simulink model "centre_out_with_two_joint_arm"  (R2021a)
settings: Solver=VariableStepAuto  StartTime=0.0  StopTime=inf  RelTol=1e-3
libraries: vrlib x1
settings Model: Creator=kbhar  LastModifiedBy=kbhar

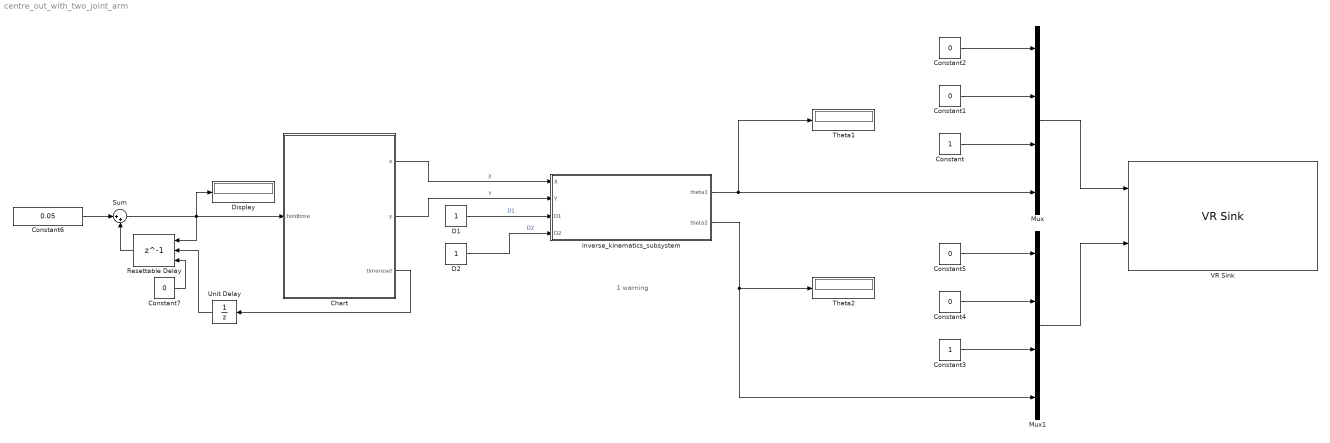
== system centre_out_with_two_joint_arm ==
  note: 1 warning
  Chart : Stateflow chart  TreatAsAtomicUnit=on
  Constant : Constant
  Constant{1..2,4..5,7} (5 alike) : Constant  Value=0
  Constant3 : Constant
  Constant6 : Constant  Value=0.05
  D1 : Constant
  D2 : Constant
  Display : Display
  Mux : Mux
  Mux1 : Mux
  Resettable Delay : Delay  DelayLength=1  InitialConditionSource=Input port  ExternalReset=Rising
      settings: InputPortMap=u0,r5,p4
  Sum : Sum  Inputs=|++
  Theta1 : Display
  Theta2 : Display
  Unit Delay : UnitDelay  SampleTime=-1  HasFrameUpgradeWarning=on
  VR Sink : vrlib/VR Sink  InstantiateOnLoad=on  SampleTime=0.1  ViewEnable=on  RemoteChange=off  RemoteView=off  FieldsWritten=shoulder_joint.rotation.4.1.1.double#elbow_joint.rotation.4.1.1.double  WorldFileName=C:\Bharat\College\Projects\Arm Control\Files\test_two_joint_arm.wrl  AutoView=off  VideoDimensions=[]  AllowVariableSize=off
  inverse_kinematics_subsystem : Subsystem
  wires:
  inverse_kinematics_subsystem/2(theta2) -> Mux1/4, Theta2/1
  inverse_kinematics_subsystem/1(theta1) -> Mux/4, Theta1/1
  Constant2/1 -> Mux/1
  Constant/1 -> Mux/3
  Constant4/1 -> Mux1/2
  Constant3/1 -> Mux1/3
  Constant5/1 -> Mux1/1
  Mux1/1 -> VR Sink/2
  Mux/1 -> VR Sink/1
  Constant1/1 -> Mux/2
  Chart/3(timereset) -> Unit Delay/1
  Constant6/1 -> Sum/1
  Resettable Delay/1 -> Sum/2
  Sum/1 -> Resettable Delay/1, Chart/1(holdtime), Display/1
  Unit Delay/1 -> Resettable Delay/2
  Chart/1(x) -> inverse_kinematics_subsystem/1(X)  "X"
  Chart/2(y) -> inverse_kinematics_subsystem/2(Y)  "Y"
  D1/1 -> inverse_kinematics_subsystem/3(D1)  "D1"
  D2/1 -> inverse_kinematics_subsystem/4(D2)  "D2"
  Constant7/1 -> Resettable Delay/3

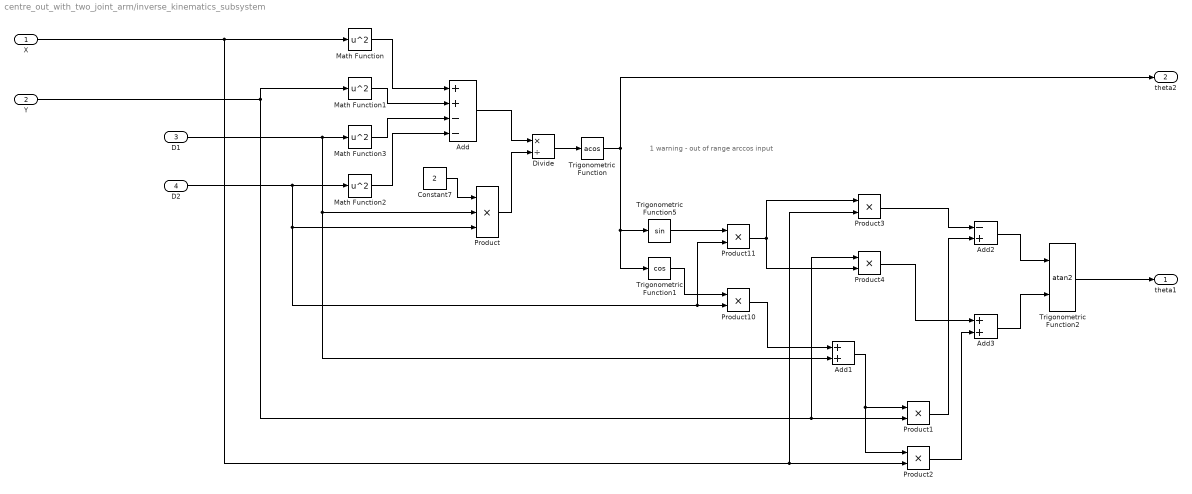
== system centre_out_with_two_joint_arm/inverse_kinematics_subsystem ==
  note: 1 warning - out of range arccos input
  X : Inport
  Y : Inport  Port=2
  D1 : Inport  Port=3
  D2 : Inport  Port=4
  Add : Sum  Inputs=++--
  Add1 : Sum
  Add2 : Sum  Inputs=-+
  Add3 : Sum
  Constant7 : Constant  Value=2
  Divide : Product  Inputs=*/
  Math Function{,1..3} (4 alike) : Math  Operator=square  SaturateOnIntegerOverflow=on
  Product : Product  Inputs=3
  Product{1..4,10..11} (6 alike) : Product
  Trigonometric Function : Trigonometry  Operator=acos  OutputSignalType=real
  Trigonometric Function1 : Trigonometry  Operator=cos
  Trigonometric Function2 : Trigonometry  Operator=atan2
  Trigonometric Function5 : Trigonometry
  theta1 : Outport
  theta2 : Outport  Port=2
  wires:
  D2/1 -> Math Function2/1, Product11/2, Product10/2, Product/3
  D1/1 -> Add1/2, Product/2, Math Function3/1
  Y/1 -> Math Function1/1, Product1/2, Product4/1
  Trigonometric Function/1 -> theta2/1, Trigonometric Function1/1, Trigonometric Function5/1
  Math Function3/1 -> Add/3
  Trigonometric Function5/1 -> Product11/1
  Product/1 -> Divide/2
  Math Function2/1 -> Add/4
  Product3/1 -> Add2/1
  Trigonometric Function1/1 -> Product10/1
  X/1 -> Product2/2, Product3/2, Math Function/1
  Math Function/1 -> Add/1
  Add1/1 -> Product1/1, Product2/1
  Constant7/1 -> Product/1
  Add3/1 -> Trigonometric Function2/2
  Product4/1 -> Add3/1
  Product1/1 -> Add2/2
  Product2/1 -> Add3/2
  Product11/1 -> Product3/1, Product4/2
  Add2/1 -> Trigonometric Function2/1
  Math Function1/1 -> Add/2
  Trigonometric Function2/1 -> theta1/1
  Add/1 -> Divide/1
  Product10/1 -> Add1/1
  Divide/1 -> Trigonometric Function/1

== stateflow chart centre_out_with_two_joint_arm/Chart ==
  state startstate
    x = 0; y = 0; timereset = 0;
  state centrestate
    x = 0; y = 0; timereset = 0;
  state resettimestate
    x = 0; y = 0; timereset = 1;
  state centrestateback
    x = 0; y = 0; timereset = 0;
  state outerstatetransition
    x = x + 0.001; y = y + 0.001; timereset = 0;
  state centrestatetransition
    x = x - 0.001; y = y - 0.001; timereset = 0;
  state outerstate
    x = sqrt(2); y = sqrt(2); timereset = 0;
  (default) -> startstate
  startstate -> centrestate
  resettimestate -> centrestate
  centrestateback -> resettimestate
  centrestate -> outerstatetransition : [holdtime>15]
  centrestatetransition -> centrestateback : [x <= 0.001 && y <=0.001]
  outerstatetransition -> outerstate : [x >= sqrt(2) - 0.001 && y >= sqrt(2) - 0.001]
  outerstate -> centrestatetransition : [holdtime>100]
  data: x output; y output; holdtime input; timereset output
